simulink model "Non_Ideal2_PV"  (R2026a)
settings: Solver=ode3  StopTime=0.6  FixedStep=0.01
libraries: simulink x1

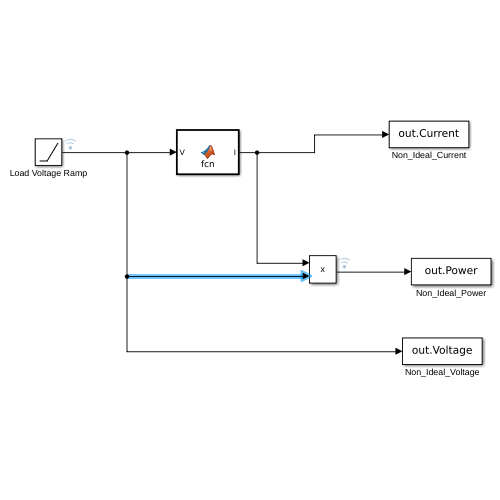
[thumbnail: Simulink's stored preview of the top-level diagram]
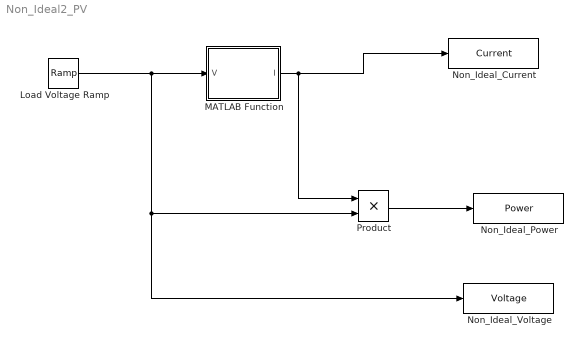
== system Non_Ideal2_PV ==
  Load Voltage Ramp : simulink/Sources/Ramp  slope=1  start=0  InitialOutput=0
  MATLAB Function : MATLAB Function  TreatAsAtomicUnit=on
  Non_Ideal_Current : ToWorkspace  VariableName=Current  SampleTime=-1
  Non_Ideal_Power : ToWorkspace  VariableName=Power  SampleTime=-1
  Non_Ideal_Voltage : ToWorkspace  VariableName=Voltage  SampleTime=-1
  Product : Product
  wires:
  Load Voltage Ramp/1 -> Non_Ideal_Voltage/1, Product/2, MATLAB Function/1(V)
  Product/1 -> Non_Ideal_Power/1
  MATLAB Function/1(I) -> Product/1, Non_Ideal_Current/1

== matlab function Non_Ideal2_PV/MATLAB Function ==
  data: V input; I output
function I = fcn(V)
% Non-ideal single-diode PV terminal current
% Solves:
% I = Isc - I0*(exp(ad*(V + I*Rs)) - 1) - (V + I*Rs)/Rp

Isc = 2.0;        % short-circuit current [A]
I0  = 5.0e-10;    % reverse saturation current [A]
ad  = 39.8;       % diode exponential constant [V^-1]
Rs  = 0.04;       % series resistance [ohm]
Rp  = 8.0;        % shunt resistance [ohm]

% Initial guess
I = Isc;

tol = 1e-8;
maxIter = 50;

for iter = 1:maxIter
    Vj = V + I*Rs;

    % Residual F(I) = 0
    F = I - Isc + I0*(exp(ad*Vj) - 1) + Vj/Rp;

    % Derivative dF/dI
    dF = 1 + I0*exp(ad*Vj)*ad*Rs + Rs/Rp;

    Inew = I - F/dF;

    if abs(Inew - I) < tol
        I = Inew;
        break;
    end

    I = Inew;
end

% Prevent nonphysical values
I = max(I,0);
I = min(I,Isc);
end
